simulink model "PTDproj"  (R2016a)
settings: Solver=ode23tb  SolverMode=SingleTasking  StartTime=0.0  StopTime=86400  RelTol=1e-4  AbsTol=1e-3
PreLoadFcn:
  | % Load Data and Parameters used by the model:
  | load power_V2G.mat
  | to=0.1;
undefined symbols (not defined in the file): A, B, C, D1, Dd, Delta, Init, j, V2G
libraries: powerlib x54, simulink x19, simulink_extras x6, sps_avr x1, V2Glib x1, powerlib_meascontrol x1
(part 2 of 3)

== system PTDproj/Scopes /Source data ==
  Complex to Magnitude-Angle : ComplexToMagnitudeAngle
  Complex to Magnitude-Angle1 : ComplexToMagnitudeAngle
  Demux : Demux  Outputs=1
  Demux1 : Demux  Outputs=1
  Gain : Gain  Gain=3/2
  Product : Product
  Product1 : Product
  Product2 : Product
  Sum : Sum  Inputs=|+-
  Trigonometric Function : Trigonometry  Operator=cos
  Trigonometric Function1 : Trigonometry
  V src : Outport
  I src : Outport  Port=2
  S src : Outport  Port=3
  P src : Outport  Port=4
  Q src : Outport  Port=5
  tag scope: P_src=global, Q_src=global, S_src=global
  wires:
  Product2/1 -> [Q_src], Q src/1
  Product1/1 -> P src/1, [P_src]
  Trigonometric Function/1 -> Product1/2
  Trigonometric Function1/1 -> Product2/2
  Sum/1 -> Trigonometric Function/1, Trigonometric Function1/1
  Complex to Magnitude-Angle/2 -> Sum/1
  [Iabc1] -> Complex to Magnitude-Angle1/1
  [Vabc1] -> Complex to Magnitude-Angle/1
  Complex to Magnitude-Angle1/2 -> Sum/2
  Product/1 -> Product1/1, Product2/1, S src/1, [S_src]
  Demux1/1 -> Product/2
  Gain/1 -> Product/1
  Complex to Magnitude-Angle1/1 -> Demux1/1, I src/1
  Complex to Magnitude-Angle/1 -> Demux/1, V src/1
  Demux/1 -> Gain/1

== system PTDproj/Scopes /Wind farm data ==
  Complex to Magnitude-Angle : ComplexToMagnitudeAngle
  Complex to Magnitude-Angle1 : ComplexToMagnitudeAngle
  Demux : Demux  Outputs=1
  Demux1 : Demux  Outputs=1
  Gain : Gain  Gain=3/2
  Product : Product
  Product1 : Product
  Product2 : Product
  Scope : Scope
  Sum : Sum  Inputs=|+-
  Trigonometric Function : Trigonometry  Operator=cos
  Trigonometric Function1 : Trigonometry
  V wind : Outport
  I wind : Outport  Port=2
  S wind : Outport  Port=3
  P wind : Outport  Port=4
  Q wind : Outport  Port=5
  Wind : Outport  Port=6
  tag scope: P_wind=global, Q_wind=global, S_wind=global
  wires:
  Demux/1 -> Gain/1
  Complex to Magnitude-Angle/1 -> V wind/1, Demux/1
  Complex to Magnitude-Angle1/1 -> I wind/1, Demux1/1
  Gain/1 -> Product/1
  Demux1/1 -> Product/2
  Product/1 -> [S_wind], S wind/1, Product2/1, Product1/1
  Complex to Magnitude-Angle1/2 -> Scope/1, Sum/2
  [Vabcwind] -> Complex to Magnitude-Angle/1
  [Iabcwind] -> Complex to Magnitude-Angle1/1
  Complex to Magnitude-Angle/2 -> Sum/1
  Sum/1 -> Trigonometric Function1/1, Trigonometric Function/1
  Trigonometric Function1/1 -> Product2/2
  Trigonometric Function/1 -> Product1/2
  Product1/1 -> [P_wind], P wind/1
  Product2/1 -> [Q_wind], Q wind/1
  [wind] -> Wind/1

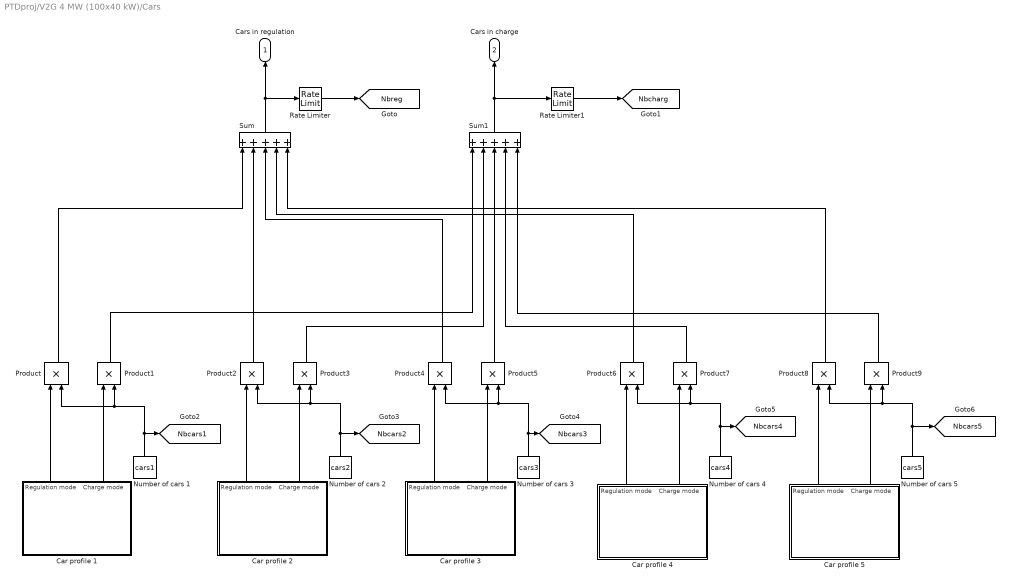
== system PTDproj/V2G 4 MW (100x40 kW)/Cars ==
  Car profile 1 : Subsystem
  Car profile 2 : Subsystem
  Car profile 3 : Subsystem
  Car profile 4 : Subsystem
  Car profile 5 : Subsystem
  Number of cars 1 : Constant  Value=cars1
  Number of cars 2 : Constant  Value=cars2
  Number of cars 3 : Constant  Value=cars3
  Number of cars 4 : Constant  Value=cars4
  Number of cars 5 : Constant  Value=cars5
  Product{,1..9} (10 alike) : Product
  Rate Limiter : RateLimiter  RisingSlewLimit=10000  FallingSlewLimit=-10000  SampleTimeMode=inherited
  Rate Limiter1 : RateLimiter  RisingSlewLimit=10000  FallingSlewLimit=-10000  SampleTimeMode=inherited
  Sum : Sum  Inputs=+++++
  Sum1 : Sum  Inputs=+++++
  Cars in regulation : Outport
  " Cars in charge" : Outport  Port=2
  tag scope: Nbcars1=global, Nbcars2=global, Nbcars3=global, Nbcars4=global, Nbcars5=global, Nbcharg=global, Nbreg=global
  wires:
  Car profile 3/2("Charge mode ") -> Product5/1
  Car profile 2/1("Regulation mode ") -> Product2/1
  Car profile 3/1("Regulation mode ") -> Product4/1
  Car profile 2/2("Charge mode ") -> Product3/1
  Car profile 4/2("Charge mode ") -> Product7/1
  Car profile 4/1("Regulation mode ") -> Product6/1
  Car profile 1/1("Regulation mode ") -> Product/1
  Car profile 1/2("Charge mode ") -> Product1/1
  Number of cars 1/1 -> Product1/2, Product/2, [Nbcars1]
  Number of cars 2/1 -> Product3/2, Product2/2, [Nbcars2]
  Number of cars 3/1 -> Product4/2, Product5/2, [Nbcars3]
  Number of cars 4/1 -> Product6/2, Product7/2, [Nbcars4]
  Number of cars 5/1 -> Product8/2, Product9/2, [Nbcars5]
  Sum/1 -> Cars in regulation/1, Rate Limiter/1
  Sum1/1 -> Rate Limiter1/1, " Cars in charge"/1
  Product/1 -> Sum/1
  Product2/1 -> Sum/2
  Product4/1 -> Sum/3
  Product6/1 -> Sum/4
  Product8/1 -> Sum/5
  Product1/1 -> Sum1/1
  Product3/1 -> Sum1/2
  Product9/1 -> Sum1/5
  Product5/1 -> Sum1/3
  Product7/1 -> Sum1/4
  Rate Limiter/1 -> [Nbreg]
  Rate Limiter1/1 -> [Nbcharg]
  Car profile 5/1("Regulation mode ") -> Product8/1
  Car profile 5/2("Charge mode ") -> Product9/1

== system PTDproj/V2G 4 MW (100x40 kW)/Charge power generation ==
  note: V1= 1/3(Vab -a^2*Vbc)
  note: S = 3* ( V * I') / 2
  note: Ia= I1
  note: Ib= a^2*I1
  S charg : Inport
  Add : Sum  Inputs=+-
  Avoid division by zero : Subsystem
  Break Alg. Loop 2 : Subsystem
  Conj1 : Math  Operator=conj  SaturateOnIntegerOverflow=on
  Demux : Demux  Outputs=2
  Gain : Gain  Gain=-1
  Product : Product  Inputs=/*  SaturateOnIntegerOverflow=on  InputSameDT=on  OutDataTypeStr=Inherit: Same as first input
  Real-Imag to Complex : RealImagToComplex
  a^2 : Gain  Gain=exp(-j*2*pi/3)  SaturateOnIntegerOverflow=on  OutDataTypeStr=Inherit: Same as input  ParamDataTypeStr=Inherit: Same as input
  "a^2 " : Gain  Gain=exp(-j*2*pi/3)  SaturateOnIntegerOverflow=on  OutDataTypeStr=Inherit: Same as input  ParamDataTypeStr=Inherit: Same as input
  a^3 : Gain  Gain=1/3  SaturateOnIntegerOverflow=on  OutDataTypeStr=Inherit: Same as input  ParamDataTypeStr=Inherit: Same as input
  a^4 : Gain  Gain=2/3  SaturateOnIntegerOverflow=on  OutDataTypeStr=Inherit: Same as input  ParamDataTypeStr=Inherit: Same as input
  tag scope: Ia2=global, Ib2=global
  wires:
  Real-Imag to Complex/1 -> Product/2
  Product/1 -> a^4/1  "I1"
  a^2/1 -> [Ib2]
  Avoid division by zero/1(O) -> Product/1  "V1"
  Conj1/1 -> Break Alg. Loop 2/1(In)
  a^3/1 -> Avoid division by zero/1(I)
  Add/1 -> a^3/1
  [Vab2] -> Add/1
  [Vbc2] -> "a^2 "/1
  "a^2 "/1 -> Add/2
  a^4/1 -> Conj1/1
  Break Alg. Loop 2/1(Out) -> [Ia2], a^2/1
  Demux/1 -> Real-Imag to Complex/1
  Demux/2 -> Real-Imag to Complex/2
  S charg/1 -> Gain/1
  Gain/1 -> Demux/1

== system PTDproj/V2G 4 MW (100x40 kW)/Grid regulation ==
  Pmax reg : Inport
  Grid regulation ocntrol : Subsystem
  Grid regulation power  generation : Subsystem
  wires:
  Grid regulation ocntrol/1(PQ) -> Grid regulation power  generation/1("PQ ")
  Pmax reg/1 -> Grid regulation ocntrol/1(Pmax reg)

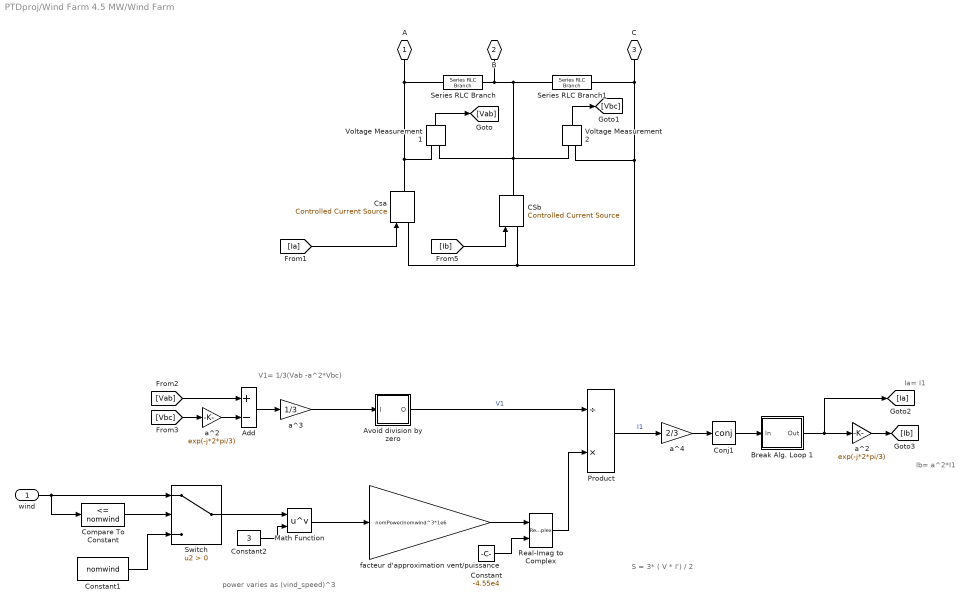
== system PTDproj/Wind Farm 4.5 MW/Wind Farm ==
  note: power varies as (vind_speed)^3
  note: V1= 1/3(Vab -a^2*Vbc)
  note: S = 3* ( V * I') / 2
  note: Ia= I1
  note: Ib= a^2*I1
  "wind " : Inport
  Add : Sum  Inputs=+-
  Avoid division by zero : Subsystem
  Break Alg. Loop 1 : Subsystem
  CSb : powerlib/Electrical Sources/Controlled Current Source  Initialize=on  Source_Type=AC  Amplitude=6286.7  Phase=(-0.5-2*pi/3)*180/pi  Frequency=60  Measurements=Current
  Compare To Constant : simulink/Logic and Bit Operations/Compare To Constant  relop=<=  const=nomwind  OutDataTypeStr=boolean
  Conj1 : Math  Operator=conj  SaturateOnIntegerOverflow=on
  Constant : Constant  Value=-4.55e4
  Constant1 : Constant  Value=nomwind
  Constant2 : Constant  Value=3
  Csa : powerlib/Electrical Sources/Controlled Current Source  Initialize=on  Source_Type=AC  Amplitude=6286.7  Phase=-0.5*180/pi  Frequency=60  Measurements=Current
  Math Function : Math  Operator=pow  SaturateOnIntegerOverflow=on
  Product : Product  Inputs=/*  SaturateOnIntegerOverflow=on  InputSameDT=on  OutDataTypeStr=Inherit: Same as first input
  Real-Imag to Complex : RealImagToComplex
  Series RLC Branch : powerlib/Elements/Series RLC Branch  LConnTagsString=__new0  RConnTagsString=__new0  BranchType=R  Resistance=1e6  Inductance=1e-3  SetiL0=off  InitialCurrent=0  Capacitance=1e-6  Setx0=off  InitialVoltage=0  Measurements=None
  Series RLC Branch1 : powerlib/Elements/Series RLC Branch  LConnTagsString=__new0  RConnTagsString=__new0  BranchType=R  Resistance=1e6  Inductance=1e-3  SetiL0=off  InitialCurrent=0  Capacitance=1e-6  Setx0=off  InitialVoltage=0  Measurements=None
  Switch : Switch  Criteria=u2 > Threshold
  Voltage Measurement1 : powerlib/Measurements/Voltage Measurement  PhasorSimulation=on  OutputType=Complex  PSBequivalent=0
  Voltage Measurement2 : powerlib/Measurements/Voltage Measurement  PhasorSimulation=on  OutputType=Complex  PSBequivalent=0
  a^2 : Gain  Gain=exp(-j*2*pi/3)  SaturateOnIntegerOverflow=on  OutDataTypeStr=Inherit: Same as input  ParamDataTypeStr=Inherit: Same as input
  "a^2 " : Gain  Gain=exp(-j*2*pi/3)  SaturateOnIntegerOverflow=on  OutDataTypeStr=Inherit: Same as input  ParamDataTypeStr=Inherit: Same as input
  a^3 : Gain  Gain=1/3  SaturateOnIntegerOverflow=on  OutDataTypeStr=Inherit: Same as input  ParamDataTypeStr=Inherit: Same as input
  a^4 : Gain  Gain=2/3  SaturateOnIntegerOverflow=on  OutDataTypeStr=Inherit: Same as input  ParamDataTypeStr=Inherit: Same as input
  facteur d'approximation vent/puissance : Gain  Gain=nomPower/nomwind^3*1e6
  A : PMIOPort  Tag=PMCPort  Port=1  Side=Right
  B : PMIOPort  Tag=PMCPort  Port=2  Side=Right
  C : PMIOPort  Tag=PMCPort  Port=3  Side=Right
  wires:
  "a^2 "/1 -> Add/2
  [Vbc] -> "a^2 "/1
  Avoid division by zero/1(O) -> Product/1  "V1"
  a^3/1 -> Avoid division by zero/1(I)
  Add/1 -> a^3/1
  [Vab] -> Add/1
  facteur d'approximation vent/puissance/1 -> Real-Imag to Complex/1
  Constant1/1 -> Switch/3
  Compare To Constant/1 -> Switch/2
  "wind "/1 -> Switch/1, Compare To Constant/1
  Constant/1 -> Real-Imag to Complex/2
  Voltage Measurement1/1 -> [Vab]
  Voltage Measurement2/1 -> [Vbc]
  Real-Imag to Complex/1 -> Product/2
  Product/1 -> a^4/1  "I1"
  a^2/1 -> [Ib]
  Conj1/1 -> Break Alg. Loop 1/1(In)
  a^4/1 -> Conj1/1
  Break Alg. Loop 1/1(Out) -> [Ia], a^2/1
  [Ib] -> CSb/1
  [Ia] -> Csa/1
  Math Function/1 -> facteur d'approximation vent/puissance/1
  Switch/1 -> Math Function/1
  Constant2/1 -> Math Function/2
  connections:
  A/RConn1 -- Csa/RConn1 -- Voltage Measurement1/LConn1 -- Series RLC Branch/LConn1
  Voltage Measurement2/LConn2 -- Series RLC Branch1/RConn1 -- C/RConn1 -- CSb/LConn1 -- Csa/LConn1
  CSb/RConn1 -- Series RLC Branch1/LConn1 -- B/RConn1 -- Series RLC Branch/RConn1 -- Voltage Measurement2/LConn1 -- Voltage Measurement1/LConn2

== system PTDproj/Wind Farm 4.5 MW/Wind control ==
  "wind " : Inport
  Compare To Constant : simulink/Logic and Bit Operations/Compare To Constant  relop=>=  const=maxwind-0.1  OutDataTypeStr=boolean  ZeroCross=off
  Compare To Constant1 : simulink/Logic and Bit Operations/Compare To Constant  relop=<=  const=nomwind  OutDataTypeStr=boolean  ZeroCross=off
  Constant1 : Constant  Value=0
  Constant2 : Constant  Value=9
  Logical Operator1 : Logic  Operator=NOT  AllPortsSameDT=off  OutDataTypeStr=boolean
  Manual Switch : ManualSwitch
  Rate Limiter2 : RateLimiter  RisingSlewLimit=1e4  FallingSlewLimit=-1e4  SampleTimeMode=inherited
  S-R Flip-Flop : simulink_extras/Flip Flops/S-R Flip-Flop  initial_condition=0
  Switch : Switch  Threshold=0.5  ZeroCross=off
  Terminator : Terminator
  Wind : Outport
  wires:
  "wind "/1 -> Switch/1, Compare To Constant/1, Compare To Constant1/1
  Constant1/1 -> Switch/3
  Logical Operator1/1 -> Switch/2
  S-R Flip-Flop/1 -> Logical Operator1/1
  Compare To Constant1/1 -> S-R Flip-Flop/2
  Compare To Constant/1 -> S-R Flip-Flop/1
  S-R Flip-Flop/2 -> Terminator/1
  Switch/1 -> Manual Switch/1
  Manual Switch/1 -> Rate Limiter2/1
  Constant2/1 -> Manual Switch/2
  Rate Limiter2/1 -> Wind/1

== system PTDproj/Load Residential = 10 MW, PF=0.15 ASM = 0.16 MVA /Residential Load/Avoid division by zero ==
  I : Inport
  Complex to Magnitude-Angle : ComplexToMagnitudeAngle
  Magnitude-Angle to Complex : MagnitudeAngleToComplex
  Saturation1 : Saturate  UpperLimit=inf  LowerLimit=1e-6
  O : Outport
  wires:
  I/1 -> Complex to Magnitude-Angle/1
  Saturation1/1 -> Magnitude-Angle to Complex/1
  Complex to Magnitude-Angle/1 -> Saturation1/1
  Magnitude-Angle to Complex/1 -> O/1
  Complex to Magnitude-Angle/2 -> Magnitude-Angle to Complex/2

== system PTDproj/Load Residential = 10 MW, PF=0.15 ASM = 0.16 MVA /Residential Load/Break Alg. Loop 1 ==
  In : Inport
  Complex to Real-Imag : ComplexToRealImag
  Real-Imag to Complex : RealImagToComplex
  imag : Subsystem  mask(Transfer Function with Initial Outputs){N=[1], D=[to  1], Y0=0, U0=0}
      mask prompts: N "Numerator:"; D "Denominator:"; Y0 "Initial output:"; U0 "Initial input:"
      mask help: Vector expressions for numerator, and denominator. Coefficients are in descending powers of s.
      mask init:
      | [A,B,C,Dd]=tf2ss(N,D);if (isempty(Y0));[m,n]=size(A);X0=zeros(1,m); end; if (isempty(U0));[m,p]=size(B);U0=zeros(1,p);end;X0=getxo(A,B,C,Dd,U0,Y0,0);
      mask Help: Specify the initial output for the transfer function.  An optimization routine attempts to determine the appropriate initial states so that the specified initial output is achieved.  For more details, see the m-file getxo.m
      mask Display: dpoly(N,D,'s')
  real : Subsystem  mask(Transfer Function with Initial Outputs){N=[1], D=[to 1], Y0=0, U0=0}
      mask prompts: N "Numerator:"; D "Denominator:"; Y0 "Initial output:"; U0 "Initial input:"
      mask help: Vector expressions for numerator, and denominator. Coefficients are in descending powers of s.
      mask init:
      | [A,B,C,Dd]=tf2ss(N,D);if (isempty(Y0));[m,n]=size(A);X0=zeros(1,m); end; if (isempty(U0));[m,p]=size(B);U0=zeros(1,p);end;X0=getxo(A,B,C,Dd,U0,Y0,0);
      mask Help: Specify the initial output for the transfer function.  An optimization routine attempts to determine the appropriate initial states so that the specified initial output is achieved.  For more details, see the m-file getxo.m
      mask Display: dpoly(N,D,'s')
  Out : Outport
  wires:
  Complex to Real-Imag/1 -> real/1(In1)
  Complex to Real-Imag/2 -> imag/1(In1)
  In/1 -> Complex to Real-Imag/1
  Real-Imag to Complex/1 -> Out/1
  real/1(Out1) -> Real-Imag to Complex/1
  imag/1(Out1) -> Real-Imag to Complex/2

== system PTDproj/Load Residential = 10 MW, PF=0.15 ASM = 0.16 MVA /Residential Load/Load ==
  1 : Constant
  Add : Sum
  Clock : Clock
  Constant : Constant
  Constant1 : Constant  Value=15/24
  Divide : Product  Inputs=*/
  Manual Switch : ManualSwitch
  Mux : Mux  Inputs=2
  P nom : Constant  Value=-nomPower*1e6
  Power consumption : Lookup_n-D  NumberOfTableDimensions=1  BreakpointsForDimension1=[1:timestep/60:24]  BeginIndexSearchUsingPreviousIndexResult=on  Table=datas  InternalRulePriority=Speed  RndMeth=Simplest  InputSameDT=on
  Power factor : Constant  Value=PF^2
  Product : Product
  Product1 : Product
  Scope : Scope
  Second-->Hour : Gain  Gain=1/(60*60)
  Sqrt : Sqrt  SaturateOnIntegerOverflow=on
  Sum : Sum  Inputs=-+
  PQ : Outport
  wires:
  Constant/1 -> Add/2
  1/1 -> Sum/1, Divide/1
  Second-->Hour/1 -> Add/1
  Sum/1 -> Sqrt/1
  Power factor/1 -> Divide/2
  Add/1 -> Power consumption/1
  P nom/1 -> Product/2
  Clock/1 -> Second-->Hour/1
  Sqrt/1 -> Product1/2
  Product/1 -> Product1/1, Mux/1
  Divide/1 -> Sum/2
  Product1/1 -> Mux/2
  Power consumption/1 -> Manual Switch/1
  Manual Switch/1 -> Product/1
  Constant1/1 -> Manual Switch/2
  Mux/1 -> Scope/1, PQ/1

== system PTDproj/PV Farm 8 MW/PV Farm/Avoid division by zero ==
  I : Inport
  Complex to Magnitude-Angle : ComplexToMagnitudeAngle
  Magnitude-Angle to Complex : MagnitudeAngleToComplex
  Saturation1 : Saturate  UpperLimit=inf  LowerLimit=1e-6
  O : Outport
  wires:
  Complex to Magnitude-Angle/2 -> Magnitude-Angle to Complex/2
  Magnitude-Angle to Complex/1 -> O/1
  Complex to Magnitude-Angle/1 -> Saturation1/1
  Saturation1/1 -> Magnitude-Angle to Complex/1
  I/1 -> Complex to Magnitude-Angle/1

== system PTDproj/PV Farm 8 MW/PV Farm/Break Alg. Loop 1 ==
  In : Inport
  Complex to Real-Imag : ComplexToRealImag
  Real-Imag to Complex : RealImagToComplex
  imag : Subsystem  mask(Transfer Function with Initial Outputs){N=[1], D=[to  1], Y0=0, U0=0}
      mask prompts: N "Numerator:"; D "Denominator:"; Y0 "Initial output:"; U0 "Initial input:"
      mask help: Vector expressions for numerator, and denominator. Coefficients are in descending powers of s.
      mask init:
      | [A,B,C,Dd]=tf2ss(N,D);if (isempty(Y0));[m,n]=size(A);X0=zeros(1,m); end; if (isempty(U0));[m,p]=size(B);U0=zeros(1,p);end;X0=getxo(A,B,C,Dd,U0,Y0,0);
      mask Help: Specify the initial output for the transfer function.  An optimization routine attempts to determine the appropriate initial states so that the specified initial output is achieved.  For more details, see the m-file getxo.m
      mask Display: dpoly(N,D,'s')
  real : Subsystem  mask(Transfer Function with Initial Outputs){N=[1], D=[to 1], Y0=0, U0=0}
      mask prompts: N "Numerator:"; D "Denominator:"; Y0 "Initial output:"; U0 "Initial input:"
      mask help: Vector expressions for numerator, and denominator. Coefficients are in descending powers of s.
      mask init:
      | [A,B,C,Dd]=tf2ss(N,D);if (isempty(Y0));[m,n]=size(A);X0=zeros(1,m); end; if (isempty(U0));[m,p]=size(B);U0=zeros(1,p);end;X0=getxo(A,B,C,Dd,U0,Y0,0);
      mask Help: Specify the initial output for the transfer function.  An optimization routine attempts to determine the appropriate initial states so that the specified initial output is achieved.  For more details, see the m-file getxo.m
      mask Display: dpoly(N,D,'s')
  Out : Outport
  wires:
  Complex to Real-Imag/1 -> real/1(In1)
  Complex to Real-Imag/2 -> imag/1(In1)
  In/1 -> Complex to Real-Imag/1
  Real-Imag to Complex/1 -> Out/1
  real/1(Out1) -> Real-Imag to Complex/1
  imag/1(Out1) -> Real-Imag to Complex/2

== system PTDproj/V2G 4 MW (100x40 kW)/Cars/Car profile 1 ==
  Add : Sum
  Charger control : Subsystem
  Clock : Clock
  Constant : Constant
  Plug state : Lookup_n-D  NumberOfTableDimensions=1  BreakpointsForDimension1=[1:24]  BeginIndexSearchUsingPreviousIndexResult=on  Table="[1 1 1 1 1 1 0 0 1 1 1 1 1 1 1 1 0 0 1 1 1 1  1 1]"  InterpMethod=Flat  InternalRulePriority=Speed  RndMeth=Simplest  InputSameDT=on
  Rate Limiter : RateLimiter  RisingSlewLimit=1e4  FallingSlewLimit=-1e4  SampleTimeMode=inherited
  Rate Limiter1 : RateLimiter  RisingSlewLimit=1e4  FallingSlewLimit=-1e4  SampleTimeMode=inherited
  SOC initialization : Lookup_n-D  NumberOfTableDimensions=1  BreakpointsForDimension1=[1:24]  BeginIndexSearchUsingPreviousIndexResult=on  Table=[0.9 0.9 0.9 0.9 0.9 0.9 -1 0.8 0.8 0.9 0.9 0.9 0.9 0.9 0.9 0.9 -1 0.8 0.8 0.9 0.9 0.9 0.9 0.9]  InterpMethod=Flat  InternalRulePriority=Speed  RndMeth=Simplest  InputSameDT=on
  Second-->Hour : Gain  Gain=1/(60*60)
  State of charge : Subsystem
  "Regulation mode " : Outport
  "Charge mode " : Outport  Port=2
  wires:
  Constant/1 -> Add/2
  Second-->Hour/1 -> Add/1
  Clock/1 -> Second-->Hour/1
  Add/1 -> SOC initialization/1, Plug state/1
  State of charge/1(SE%) -> Charger control/1(SE%)
  Charger control/1("Charge mode ") -> "Charge mode "/1, State of charge/1(charge)
  Charger control/2("Regulation mode ") -> "Regulation mode "/1
  SOC initialization/1 -> Rate Limiter/1
  Plug state/1 -> Rate Limiter1/1
  Rate Limiter/1 -> State of charge/2(SOC)
  Rate Limiter1/1 -> Charger control/2("Plug "), State of charge/3(Plug)

== system PTDproj/V2G 4 MW (100x40 kW)/Cars/Car profile 2 ==
  Add1 : Sum
  Charger control : Subsystem
  Clock1 : Clock
  Constant1 : Constant
  Plug state : Lookup_n-D  NumberOfTableDimensions=1  BreakpointsForDimension1=[1:24]  BeginIndexSearchUsingPreviousIndexResult=on  Table="[1 1 1 1 1 1 0 0 0 0 0 0 0 0 0 0 0 0 1 1 1 1  1 1]"  InterpMethod=Flat  InternalRulePriority=Speed  RndMeth=Simplest  InputSameDT=on
  Rate Limiter2 : RateLimiter  RisingSlewLimit=1e4  FallingSlewLimit=-1e4  SampleTimeMode=inherited
  Rate Limiter3 : RateLimiter  RisingSlewLimit=1e4  FallingSlewLimit=-1e4  SampleTimeMode=inherited
  SOC initialization : Lookup_n-D  NumberOfTableDimensions=1  BreakpointsForDimension1=[1:24]  BeginIndexSearchUsingPreviousIndexResult=on  Table=[0.9 0.9 0.9 0.9 0.9 0.9 -1 0.8 0.8 0.9 0.9 0.9 0.9 0.9 0.9 0.9 -1 0.8 0.6 0.9 0.9 0.9 0.9 0.9]  InterpMethod=Flat  InternalRulePriority=Speed  RndMeth=Simplest  InputSameDT=on
  Second-->Hour1 : Gain  Gain=1/(60*60)
  State of charge : Subsystem
  "Regulation mode " : Outport
  "Charge mode " : Outport  Port=2
  wires:
  Constant1/1 -> Add1/2
  Second-->Hour1/1 -> Add1/1
  Clock1/1 -> Second-->Hour1/1
  Add1/1 -> Plug state/1, SOC initialization/1
  State of charge/1(SE%) -> Charger control/1(SE%)
  Charger control/1("Charge mode ") -> State of charge/1(charge), "Charge mode "/1
  Charger control/2("Regulation mode ") -> "Regulation mode "/1
  SOC initialization/1 -> Rate Limiter2/1
  Plug state/1 -> Rate Limiter3/1
  Rate Limiter2/1 -> State of charge/2(SOC)
  Rate Limiter3/1 -> Charger control/2("Plug "), State of charge/3(Plug)

== system PTDproj/V2G 4 MW (100x40 kW)/Cars/Car profile 3 ==
  Add1 : Sum
  Charger control : Subsystem
  Clock1 : Clock
  Constant1 : Constant
  Plug state : Lookup_n-D  NumberOfTableDimensions=1  BreakpointsForDimension1=[1:24]  BeginIndexSearchUsingPreviousIndexResult=on  Table="[1 1 1 1 1 0 0 0 1 1 1 1 1 1 1 1 0 0 0 1 1 1  1 1]"  InterpMethod=Flat  InternalRulePriority=Speed  RndMeth=Simplest  InputSameDT=on
  Rate Limiter2 : RateLimiter  RisingSlewLimit=1e4  FallingSlewLimit=-1e4  SampleTimeMode=inherited
  Rate Limiter3 : RateLimiter  RisingSlewLimit=1e4  FallingSlewLimit=-1e4  SampleTimeMode=inherited
  SOC initialization : Lookup_n-D  NumberOfTableDimensions=1  BreakpointsForDimension1=[1:24]  BeginIndexSearchUsingPreviousIndexResult=on  Table=[0.9 0.9 0.9 0.9 0.9 -1 -1 0.7 0.7 0.9 0.9 0.9 0.9 0.9 0.9 0.9 -1 0.8 0.7 0.9 0.9 0.9 0.9 0.9]  InterpMethod=Flat  InternalRulePriority=Speed  RndMeth=Simplest  InputSameDT=on
  Second-->Hour1 : Gain  Gain=1/(60*60)
  State of charge : Subsystem
  "Regulation mode " : Outport
  "Charge mode " : Outport  Port=2
  wires:
  Constant1/1 -> Add1/2
  Second-->Hour1/1 -> Add1/1
  Clock1/1 -> Second-->Hour1/1
  Add1/1 -> Plug state/1, SOC initialization/1
  Charger control/1("Charge mode ") -> State of charge/1(charge), "Charge mode "/1
  Charger control/2("Regulation mode ") -> "Regulation mode "/1
  SOC initialization/1 -> Rate Limiter2/1
  Plug state/1 -> Rate Limiter3/1
  Rate Limiter2/1 -> State of charge/2(SOC)
  Rate Limiter3/1 -> State of charge/3(Plug), Charger control/2("Plug ")
  State of charge/1(SE%) -> Charger control/1(SE%)

== system PTDproj/V2G 4 MW (100x40 kW)/Cars/Car profile 4 ==
  Add1 : Sum
  Charger control : Subsystem
  Clock1 : Clock
  Constant1 : Constant
  Plug state : Lookup_n-D  NumberOfTableDimensions=1  BreakpointsForDimension1=[1:24]  BeginIndexSearchUsingPreviousIndexResult=on  Table="[1 1 1 1 1 1 1 1 1 1 1 1 1 1 1 1 1 1 1 1 1 1  1 1]"  InterpMethod=Flat  InternalRulePriority=Speed  RndMeth=Simplest  InputSameDT=on
  Rate Limiter2 : RateLimiter  RisingSlewLimit=1e4  FallingSlewLimit=-1e4  SampleTimeMode=inherited
  Rate Limiter3 : RateLimiter  RisingSlewLimit=1e4  FallingSlewLimit=-1e4  SampleTimeMode=inherited
  SOC initialization : Lookup_n-D  NumberOfTableDimensions=1  BreakpointsForDimension1=[1:24]  BeginIndexSearchUsingPreviousIndexResult=on  Table=[0.9 0.9 0.9 0.9 0.9 0.9 0.8 0.8 0.8 0.9 0.9 0.9 0.9 0.9 0.9 0.9 0.8 0.8 0.8 0.9 0.9 0.9 0.9 0.9]  InterpMethod=Flat  InternalRulePriority=Speed  RndMeth=Simplest  InputSameDT=on
  Second-->Hour1 : Gain  Gain=1/(60*60)
  State of charge : Subsystem
  "Regulation mode " : Outport
  "Charge mode " : Outport  Port=2
  wires:
  Constant1/1 -> Add1/2
  Second-->Hour1/1 -> Add1/1
  Clock1/1 -> Second-->Hour1/1
  Add1/1 -> Plug state/1, SOC initialization/1
  State of charge/1(SE%) -> Charger control/1(SE%)
  Charger control/1("Charge mode ") -> State of charge/1(charge), "Charge mode "/1
  Charger control/2("Regulation mode ") -> "Regulation mode "/1
  SOC initialization/1 -> Rate Limiter2/1
  Plug state/1 -> Rate Limiter3/1
  Rate Limiter2/1 -> State of charge/2(SOC)
  Rate Limiter3/1 -> Charger control/2("Plug "), State of charge/3(Plug)

== system PTDproj/V2G 4 MW (100x40 kW)/Cars/Car profile 5 ==
  Add : Sum
  Charger control : Subsystem
  Clock : Clock
  Constant : Constant
  Plug state : Lookup_n-D  NumberOfTableDimensions=1  BreakpointsForDimension1=[1:24]  BeginIndexSearchUsingPreviousIndexResult=on  Table="[0 0 0 0 1 1 1 1 1 1 1 1 1 1 1 1 1 1 1 1 0 0  0 0]"  InterpMethod=Flat  InternalRulePriority=Speed  RndMeth=Simplest  InputSameDT=on
  Rate Limiter : RateLimiter  RisingSlewLimit=1e4  FallingSlewLimit=-1e4  SampleTimeMode=inherited
  Rate Limiter1 : RateLimiter  RisingSlewLimit=1e4  FallingSlewLimit=-1e4  SampleTimeMode=inherited
  SOC initialization : Lookup_n-D  NumberOfTableDimensions=1  BreakpointsForDimension1=[1:24]  BeginIndexSearchUsingPreviousIndexResult=on  Table=[-1 0.9 0.7 0.7 0.7 0.8 0.8 0.8 0.8 0.8 0.9 0.9 0.9 0.9 0.9 0.9 0.8 0.8 0.8 0.9 -1 0.9 0.9 0.9]  InterpMethod=Flat  InternalRulePriority=Speed  RndMeth=Simplest  InputSameDT=on
  Second-->Hour : Gain  Gain=1/(60*60)
  State of charge : Subsystem
  "Regulation mode " : Outport
  "Charge mode " : Outport  Port=2
  wires:
  Rate Limiter1/1 -> State of charge/1(Plug), Charger control/2("Plug ")
  Rate Limiter/1 -> State of charge/2(SOC)
  Plug state/1 -> Rate Limiter1/1
  SOC initialization/1 -> Rate Limiter/1
  Charger control/2("Regulation mode ") -> "Regulation mode "/1
  Charger control/1("Charge mode ") -> "Charge mode "/1, State of charge/3(charge)
  State of charge/1(SE%) -> Charger control/1(SE%)
  Add/1 -> Plug state/1, SOC initialization/1
  Clock/1 -> Second-->Hour/1
  Second-->Hour/1 -> Add/1
  Constant/1 -> Add/2

== system PTDproj/V2G 4 MW (100x40 kW)/Charge power generation/Avoid division by zero ==
  I : Inport
  Complex to Magnitude-Angle : ComplexToMagnitudeAngle
  Magnitude-Angle to Complex : MagnitudeAngleToComplex
  Saturation1 : Saturate  UpperLimit=inf  LowerLimit=1e-6
  O : Outport
  wires:
  I/1 -> Complex to Magnitude-Angle/1
  Saturation1/1 -> Magnitude-Angle to Complex/1
  Complex to Magnitude-Angle/1 -> Saturation1/1
  Magnitude-Angle to Complex/1 -> O/1
  Complex to Magnitude-Angle/2 -> Magnitude-Angle to Complex/2

== system PTDproj/V2G 4 MW (100x40 kW)/Charge power generation/Break Alg. Loop 2 ==
  In : Inport
  Complex to Real-Imag : ComplexToRealImag
  Real-Imag to Complex : RealImagToComplex
  imag : Subsystem  mask(Transfer Function with Initial Outputs){N=[1], D=[to  1], Y0=0, U0=0}
      mask prompts: N "Numerator:"; D "Denominator:"; Y0 "Initial output:"; U0 "Initial input:"
      mask help: Vector expressions for numerator, and denominator. Coefficients are in descending powers of s.
      mask init:
      | [A,B,C,Dd]=tf2ss(N,D);if (isempty(Y0));[m,n]=size(A);X0=zeros(1,m); end; if (isempty(U0));[m,p]=size(B);U0=zeros(1,p);end;X0=getxo(A,B,C,Dd,U0,Y0,0);
      mask Help: Specify the initial output for the transfer function.  An optimization routine attempts to determine the appropriate initial states so that the specified initial output is achieved.  For more details, see the m-file getxo.m
      mask Display: dpoly(N,D,'s')
  real : Subsystem  mask(Transfer Function with Initial Outputs){N=[1], D=[to 1], Y0=0, U0=0}
      mask prompts: N "Numerator:"; D "Denominator:"; Y0 "Initial output:"; U0 "Initial input:"
      mask help: Vector expressions for numerator, and denominator. Coefficients are in descending powers of s.
      mask init:
      | [A,B,C,Dd]=tf2ss(N,D);if (isempty(Y0));[m,n]=size(A);X0=zeros(1,m); end; if (isempty(U0));[m,p]=size(B);U0=zeros(1,p);end;X0=getxo(A,B,C,Dd,U0,Y0,0);
      mask Help: Specify the initial output for the transfer function.  An optimization routine attempts to determine the appropriate initial states so that the specified initial output is achieved.  For more details, see the m-file getxo.m
      mask Display: dpoly(N,D,'s')
  Out : Outport
  wires:
  Complex to Real-Imag/1 -> real/1(In1)
  Complex to Real-Imag/2 -> imag/1(In1)
  In/1 -> Complex to Real-Imag/1
  Real-Imag to Complex/1 -> Out/1
  real/1(Out1) -> Real-Imag to Complex/1
  imag/1(Out1) -> Real-Imag to Complex/2

== system PTDproj/V2G 4 MW (100x40 kW)/Grid regulation/Grid regulation ocntrol ==
  Pmax reg : Inport
  Clock : Clock
  Compare To Constant : simulink/Logic and Bit Operations/Compare To Constant  relop=>=  const=5e-4  OutDataTypeStr=boolean  ZeroCross=off
  Compare To Constant1 : simulink/Logic and Bit Operations/Compare To Constant  relop=<=  const=-5e-4  OutDataTypeStr=boolean  ZeroCross=off
  Compare To Constant2 : simulink/Logic and Bit Operations/Compare To Constant  relop=>  const=1  OutDataTypeStr=boolean  ZeroCross=off
  Derivative : Derivative
  Gain : Gain  Gain=regGain(2)*1e6
  Gain1 : Gain  Gain=regGain(1)*1e6
  Gain2 : Gain  Gain=-1
  Integrator Limited : Integrator  ExternalReset=falling  UpperSaturationLimit=1e6  LowerSaturationLimit=-1e6
  Logical Operator : Logic  Operator=OR  AllPortsSameDT=off  OutDataTypeStr=boolean
  Logical Operator1 : Logic  AllPortsSameDT=off  OutDataTypeStr=boolean
  Mux : Mux  Inputs=2
  Q : Constant  Value=0
  Q1 : Constant  Value=0
  Saturation Dynamic : simulink/Discontinuities/Saturation Dynamic  OutMin=[]  OutMax=[]  OutDataTypeStr=Inherit: Same as second input  OutDataType=fixdt(1, 16)  OutScaling=2^-10  DoSatur=off
  Sum : Sum  Inputs=|+-
  Sum1 : Sum  Inputs=|++
  Switch : Switch  Threshold=0.5  ZeroCross=off
  wref : Constant
  PQ : Outport
  wires:
  Compare To Constant2/1 -> Logical Operator1/2
  Clock/1 -> Compare To Constant2/1
  Logical Operator/1 -> Logical Operator1/1
  Gain2/1 -> Saturation Dynamic/3
  Pmax reg/1 -> Saturation Dynamic/1, Gain2/1
  Integrator Limited/1 -> Saturation Dynamic/2
  Compare To Constant1/1 -> Logical Operator/2
  Compare To Constant/1 -> Logical Operator/1
  Sum/1 -> Compare To Constant/1, Compare To Constant1/1, Switch/1
  Switch/1 -> Derivative/1, Gain/1
  Gain/1 -> Sum1/2
  Gain1/1 -> Sum1/1
  Derivative/1 -> Gain1/1
  Sum1/1 -> Integrator Limited/1
  Q1/1 -> Switch/3
  [wm] -> Sum/2
  wref/1 -> Sum/1
  Q/1 -> Mux/2
  Mux/1 -> PQ/1
  Logical Operator1/1 -> Integrator Limited/2, Switch/2
  Saturation Dynamic/1 -> Mux/1

== system PTDproj/V2G 4 MW (100x40 kW)/Grid regulation/Grid regulation power  generation ==
  note: V1= 1/3(Vab -a^2*Vbc)
  note: S = 3* ( V * I') / 2
  note: Ia= I1
  note: Ib= a^2*I1
  "PQ " : Inport
  Add : Sum  Inputs=+-
  Avoid division by zero : Subsystem
  Break Alg. Loop 1 : Subsystem
  Conj1 : Math  Operator=conj  SaturateOnIntegerOverflow=on
  Demux : Demux  Outputs=2
  Product : Product  Inputs=/*  SaturateOnIntegerOverflow=on  InputSameDT=on  OutDataTypeStr=Inherit: Same as first input
  Real-Imag to Complex : RealImagToComplex
  a^2 : Gain  Gain=exp(-j*2*pi/3)  SaturateOnIntegerOverflow=on  OutDataTypeStr=Inherit: Same as input  ParamDataTypeStr=Inherit: Same as input
  "a^2 " : Gain  Gain=exp(-j*2*pi/3)  SaturateOnIntegerOverflow=on  OutDataTypeStr=Inherit: Same as input  ParamDataTypeStr=Inherit: Same as input
  a^3 : Gain  Gain=1/3  SaturateOnIntegerOverflow=on  OutDataTypeStr=Inherit: Same as input  ParamDataTypeStr=Inherit: Same as input
  a^4 : Gain  Gain=2/3  SaturateOnIntegerOverflow=on  OutDataTypeStr=Inherit: Same as input  ParamDataTypeStr=Inherit: Same as input
  tag scope: Ia1=global, Ib1=global
  wires:
  Real-Imag to Complex/1 -> Product/2
  Product/1 -> a^4/1  "I1"
  Avoid division by zero/1(O) -> Product/1  "V1"
  Conj1/1 -> Break Alg. Loop 1/1(In)
  a^3/1 -> Avoid division by zero/1(I)
  Add/1 -> a^3/1
  [Vab1] -> Add/1
  [Vbc1] -> "a^2 "/1
  "a^2 "/1 -> Add/2
  a^4/1 -> Conj1/1
  Break Alg. Loop 1/1(Out) -> [Ia1], a^2/1
  Demux/1 -> Real-Imag to Complex/1
  Demux/2 -> Real-Imag to Complex/2
  "PQ "/1 -> Demux/1
  a^2/1 -> [Ib1]

== system PTDproj/Wind Farm 4.5 MW/Wind Farm/Avoid division by zero ==
  I : Inport
  Complex to Magnitude-Angle : ComplexToMagnitudeAngle
  Magnitude-Angle to Complex : MagnitudeAngleToComplex
  Saturation1 : Saturate  UpperLimit=inf  LowerLimit=1e-6
  O : Outport
  wires:
  I/1 -> Complex to Magnitude-Angle/1
  Saturation1/1 -> Magnitude-Angle to Complex/1
  Complex to Magnitude-Angle/1 -> Saturation1/1
  Magnitude-Angle to Complex/1 -> O/1
  Complex to Magnitude-Angle/2 -> Magnitude-Angle to Complex/2

== system PTDproj/Wind Farm 4.5 MW/Wind Farm/Break Alg. Loop 1 ==
  In : Inport
  Complex to Real-Imag : ComplexToRealImag
  Real-Imag to Complex : RealImagToComplex
  imag : Subsystem  mask(Transfer Function with Initial Outputs){N=[1], D=[to  1], Y0=0, U0=0}
      mask prompts: N "Numerator:"; D "Denominator:"; Y0 "Initial output:"; U0 "Initial input:"
      mask help: Vector expressions for numerator, and denominator. Coefficients are in descending powers of s.
      mask init:
      | [A,B,C,Dd]=tf2ss(N,D);if (isempty(Y0));[m,n]=size(A);X0=zeros(1,m); end; if (isempty(U0));[m,p]=size(B);U0=zeros(1,p);end;X0=getxo(A,B,C,Dd,U0,Y0,0);
      mask Help: Specify the initial output for the transfer function.  An optimization routine attempts to determine the appropriate initial states so that the specified initial output is achieved.  For more details, see the m-file getxo.m
      mask Display: dpoly(N,D,'s')
  real : Subsystem  mask(Transfer Function with Initial Outputs){N=[1], D=[to 1], Y0=0, U0=0}
      mask prompts: N "Numerator:"; D "Denominator:"; Y0 "Initial output:"; U0 "Initial input:"
      mask help: Vector expressions for numerator, and denominator. Coefficients are in descending powers of s.
      mask init:
      | [A,B,C,Dd]=tf2ss(N,D);if (isempty(Y0));[m,n]=size(A);X0=zeros(1,m); end; if (isempty(U0));[m,p]=size(B);U0=zeros(1,p);end;X0=getxo(A,B,C,Dd,U0,Y0,0);
      mask Help: Specify the initial output for the transfer function.  An optimization routine attempts to determine the appropriate initial states so that the specified initial output is achieved.  For more details, see the m-file getxo.m
      mask Display: dpoly(N,D,'s')
  Out : Outport
  wires:
  In/1 -> Complex to Real-Imag/1
  Real-Imag to Complex/1 -> Out/1
  real/1(Out1) -> Real-Imag to Complex/1
  imag/1(Out1) -> Real-Imag to Complex/2
  Complex to Real-Imag/2 -> imag/1(In1)
  Complex to Real-Imag/1 -> real/1(In1)

== system PTDproj/Load Residential = 10 MW, PF=0.15 ASM = 0.16 MVA /Residential Load/Break Alg. Loop 1/imag ==
  In1 : Inport
  State Space : StateSpace  A=A  B=B  C=C  D=Dd  X0=X0
  Out1 : Outport  InitialOutput=0
  wires:
  State Space/1 -> Out1/1
  In1/1 -> State Space/1

== system PTDproj/Load Residential = 10 MW, PF=0.15 ASM = 0.16 MVA /Residential Load/Break Alg. Loop 1/real ==
  In1 : Inport
  State Space : StateSpace  A=A  B=B  C=C  D=Dd  X0=X0
  Out1 : Outport  InitialOutput=0
  wires:
  State Space/1 -> Out1/1
  In1/1 -> State Space/1

== system PTDproj/PV Farm 8 MW/PV Farm/Break Alg. Loop 1/imag ==
  In1 : Inport
  State Space : StateSpace  A=A  B=B  C=C  D=Dd  X0=X0
  Out1 : Outport  InitialOutput=0
  wires:
  State Space/1 -> Out1/1
  In1/1 -> State Space/1

== system PTDproj/PV Farm 8 MW/PV Farm/Break Alg. Loop 1/real ==
  In1 : Inport
  State Space : StateSpace  A=A  B=B  C=C  D=Dd  X0=X0
  Out1 : Outport  InitialOutput=0
  wires:
  State Space/1 -> Out1/1
  In1/1 -> State Space/1

== system PTDproj/V2G 4 MW (100x40 kW)/Cars/Car profile 1/Charger control ==
  SE% : Inport
  "Plug " : Inport  Port=2
  Compare To Constant : simulink/Logic and Bit Operations/Compare To Constant  relop=<=  const=85  OutDataTypeStr=boolean  ZeroCross=off
  Compare To Constant1 : simulink/Logic and Bit Operations/Compare To Constant  relop=>=  const=95  OutDataTypeStr=boolean  ZeroCross=off
  Logical Operator : Logic  AllPortsSameDT=off  OutDataTypeStr=boolean
  Logical Operator1 : Logic  Operator=NOT  AllPortsSameDT=off  OutDataTypeStr=boolean
  Logical Operator2 : Logic  AllPortsSameDT=off  OutDataTypeStr=boolean
  S-R Flip-Flop : simulink_extras/Flip Flops/S-R Flip-Flop  initial_condition=0
  Terminator : Terminator
  "Charge mode " : Outport
  "Regulation mode " : Outport  Port=2
  wires:
  SE%/1 -> Compare To Constant/1, Compare To Constant1/1
  Compare To Constant/1 -> S-R Flip-Flop/1
  Compare To Constant1/1 -> S-R Flip-Flop/2
  "Plug "/1 -> Logical Operator2/2, Logical Operator/2
  S-R Flip-Flop/1 -> Logical Operator/1, Logical Operator1/1
  Logical Operator/1 -> "Charge mode "/1
  Logical Operator2/1 -> "Regulation mode "/1
  Logical Operator1/1 -> Logical Operator2/1
  S-R Flip-Flop/2 -> Terminator/1

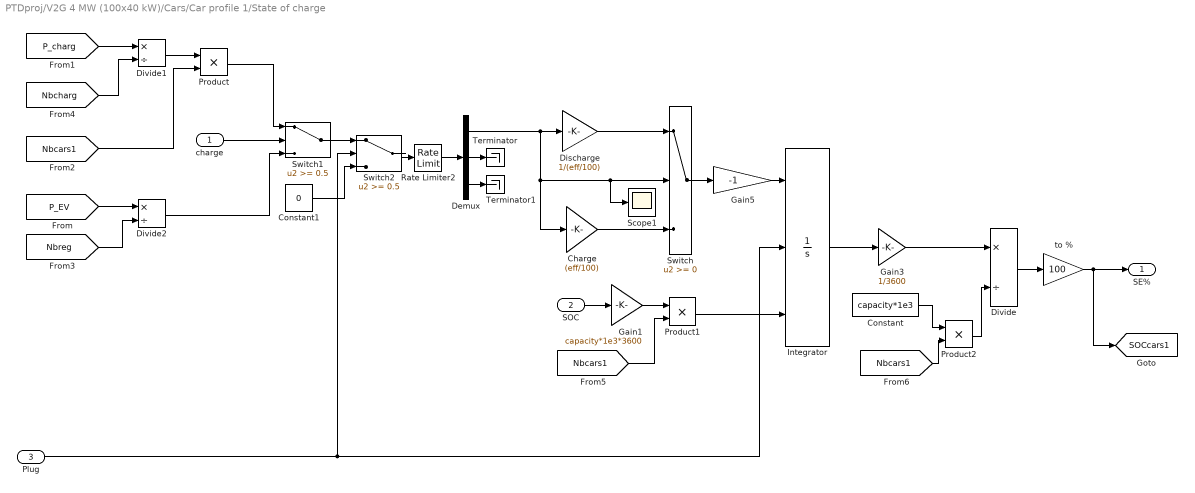
== system PTDproj/V2G 4 MW (100x40 kW)/Cars/Car profile 1/State of charge ==
  charge : Inport
  SOC : Inport  Port=2
  Plug : Inport  Port=3
  Charge : Gain  Gain=(eff/100)
  Constant : Constant  Value=capacity*1e3
  Constant1 : Constant  Value=0
  Demux : Demux  Outputs=3
  Discharge : Gain  Gain=1/(eff/100)
  Divide : Product  Inputs=*/
  Divide1 : Product  Inputs=*/
  Divide2 : Product  Inputs=*/
  Gain1 : Gain  Gain=capacity*1e3*3600
  Gain3 : Gain  Gain=1/3600
  Gain5 : Gain  Gain=-1
  Integrator : Integrator  ExternalReset=either  InitialConditionSource=external  InitialCondition=Init*850e3*3600
  Product : Product
  Product1 : Product
  Product2 : Product
  Rate Limiter2 : RateLimiter  RisingSlewLimit=1e4  FallingSlewLimit=-1e4  SampleTimeMode=inherited
  Scope1 : Scope
  Switch : Switch  ZeroCross=off
  Switch1 : Switch  Threshold=0.5  ZeroCross=off
  Switch2 : Switch  Threshold=0.5  ZeroCross=off
  Terminator : Terminator
  Terminator1 : Terminator
  to % : Gain  Gain=100
  SE% : Outport
  tag scope: SOCcars1=global
  wires:
  Discharge/1 -> Switch/1
  Charge/1 -> Switch/3
  Switch/1 -> Gain5/1
  Gain5/1 -> Integrator/1
  Integrator/1 -> Gain3/1
  Divide/1 -> to %/1
  Gain3/1 -> Divide/1
  to %/1 -> [SOCcars1], SE%/1
  Demux/2 -> Terminator/1
  Demux/3 -> Terminator1/1
  Plug/1 -> Integrator/2, Switch2/2
  SOC/1 -> Gain1/1
  charge/1 -> Switch1/2
  Demux/1 -> Charge/1, Scope1/1, Switch/2, Discharge/1
  [P_charg] -> Divide1/1
  [Nbreg] -> Divide2/2
  [P_EV] -> Divide2/1
  [Nbcharg] -> Divide1/2
  Divide1/1 -> Product/1
  [Nbcars1] -> Product/2
  Product/1 -> Switch1/1
  Divide2/1 -> Switch1/3
  Switch1/1 -> Switch2/1
  Constant1/1 -> Switch2/3
  Switch2/1 -> Rate Limiter2/1
  [Nbcars1] -> Product1/2
  Gain1/1 -> Product1/1
  Product1/1 -> Integrator/3
  Product2/1 -> Divide/2
  [Nbcars1] -> Product2/2
  Constant/1 -> Product2/1
  Rate Limiter2/1 -> Demux/1

== system PTDproj/V2G 4 MW (100x40 kW)/Cars/Car profile 2/Charger control ==
  SE% : Inport
  "Plug " : Inport  Port=2
  Compare To Constant : simulink/Logic and Bit Operations/Compare To Constant  relop=<=  const=85  OutDataTypeStr=boolean  ZeroCross=off
  Compare To Constant1 : simulink/Logic and Bit Operations/Compare To Constant  relop=>=  const=95  OutDataTypeStr=boolean  ZeroCross=off
  Logical Operator : Logic  AllPortsSameDT=off  OutDataTypeStr=boolean
  Logical Operator1 : Logic  Operator=NOT  AllPortsSameDT=off  OutDataTypeStr=boolean
  Logical Operator2 : Logic  AllPortsSameDT=off  OutDataTypeStr=boolean
  S-R Flip-Flop : simulink_extras/Flip Flops/S-R Flip-Flop  initial_condition=0
  Terminator : Terminator
  "Charge mode " : Outport
  "Regulation mode " : Outport  Port=2
  wires:
  SE%/1 -> Compare To Constant/1, Compare To Constant1/1
  Compare To Constant/1 -> S-R Flip-Flop/1
  Compare To Constant1/1 -> S-R Flip-Flop/2
  "Plug "/1 -> Logical Operator2/2, Logical Operator/2
  S-R Flip-Flop/1 -> Logical Operator/1, Logical Operator1/1
  Logical Operator/1 -> "Charge mode "/1
  Logical Operator2/1 -> "Regulation mode "/1
  Logical Operator1/1 -> Logical Operator2/1
  S-R Flip-Flop/2 -> Terminator/1

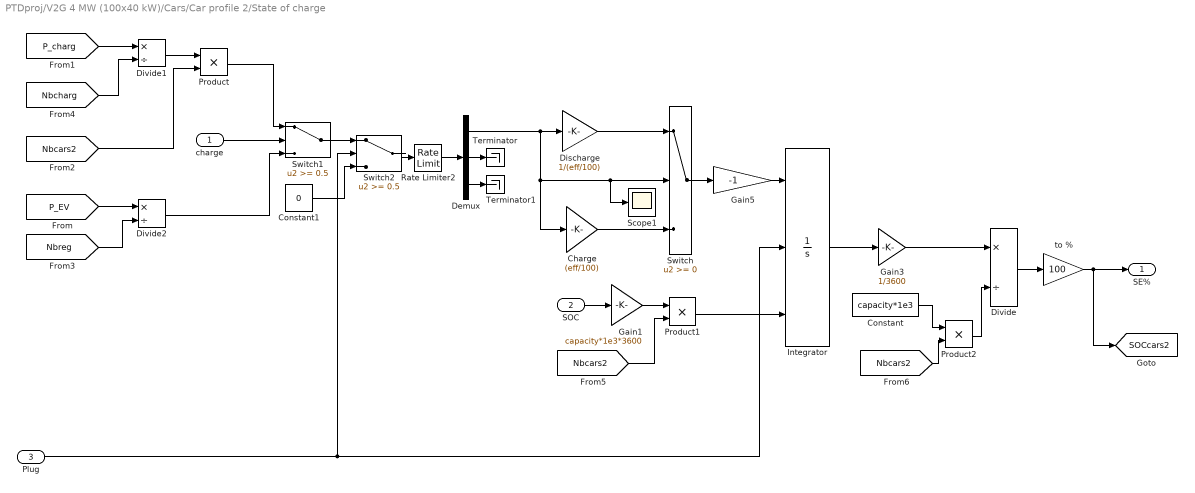
== system PTDproj/V2G 4 MW (100x40 kW)/Cars/Car profile 2/State of charge ==
  charge : Inport
  SOC : Inport  Port=2
  Plug : Inport  Port=3
  Charge : Gain  Gain=(eff/100)
  Constant : Constant  Value=capacity*1e3
  Constant1 : Constant  Value=0
  Demux : Demux  Outputs=3
  Discharge : Gain  Gain=1/(eff/100)
  Divide : Product  Inputs=*/
  Divide1 : Product  Inputs=*/
  Divide2 : Product  Inputs=*/
  Gain1 : Gain  Gain=capacity*1e3*3600
  Gain3 : Gain  Gain=1/3600
  Gain5 : Gain  Gain=-1
  Integrator : Integrator  ExternalReset=either  InitialConditionSource=external  InitialCondition=Init*850e3*3600
  Product : Product
  Product1 : Product
  Product2 : Product
  Rate Limiter2 : RateLimiter  RisingSlewLimit=1e4  FallingSlewLimit=-1e4  SampleTimeMode=inherited
  Scope1 : Scope
  Switch : Switch  ZeroCross=off
  Switch1 : Switch  Threshold=0.5  ZeroCross=off
  Switch2 : Switch  Threshold=0.5  ZeroCross=off
  Terminator : Terminator
  Terminator1 : Terminator
  to % : Gain  Gain=100
  SE% : Outport
  tag scope: SOCcars2=global
  wires:
  Discharge/1 -> Switch/1
  Charge/1 -> Switch/3
  Switch/1 -> Gain5/1
  Gain5/1 -> Integrator/1
  Integrator/1 -> Gain3/1
  Divide/1 -> to %/1
  Gain3/1 -> Divide/1
  to %/1 -> [SOCcars2], SE%/1
  Demux/2 -> Terminator/1
  Demux/3 -> Terminator1/1
  Plug/1 -> Integrator/2, Switch2/2
  SOC/1 -> Gain1/1
  charge/1 -> Switch1/2
  Demux/1 -> Charge/1, Scope1/1, Switch/2, Discharge/1
  [P_charg] -> Divide1/1
  [Nbreg] -> Divide2/2
  [P_EV] -> Divide2/1
  [Nbcharg] -> Divide1/2
  Divide1/1 -> Product/1
  [Nbcars2] -> Product/2
  Product/1 -> Switch1/1
  Divide2/1 -> Switch1/3
  Switch1/1 -> Switch2/1
  Constant1/1 -> Switch2/3
  Switch2/1 -> Rate Limiter2/1
  [Nbcars2] -> Product1/2
  Gain1/1 -> Product1/1
  Product1/1 -> Integrator/3
  Product2/1 -> Divide/2
  [Nbcars2] -> Product2/2
  Constant/1 -> Product2/1
  Rate Limiter2/1 -> Demux/1

== system PTDproj/V2G 4 MW (100x40 kW)/Cars/Car profile 3/Charger control ==
  SE% : Inport
  "Plug " : Inport  Port=2
  Compare To Constant : simulink/Logic and Bit Operations/Compare To Constant  relop=<=  const=85  OutDataTypeStr=boolean  ZeroCross=off
  Compare To Constant1 : simulink/Logic and Bit Operations/Compare To Constant  relop=>=  const=95  OutDataTypeStr=boolean  ZeroCross=off
  Logical Operator : Logic  AllPortsSameDT=off  OutDataTypeStr=boolean
  Logical Operator1 : Logic  Operator=NOT  AllPortsSameDT=off  OutDataTypeStr=boolean
  Logical Operator2 : Logic  AllPortsSameDT=off  OutDataTypeStr=boolean
  S-R Flip-Flop : simulink_extras/Flip Flops/S-R Flip-Flop  initial_condition=0
  Terminator : Terminator
  "Charge mode " : Outport
  "Regulation mode " : Outport  Port=2
  wires:
  SE%/1 -> Compare To Constant/1, Compare To Constant1/1
  Compare To Constant/1 -> S-R Flip-Flop/1
  Compare To Constant1/1 -> S-R Flip-Flop/2
  "Plug "/1 -> Logical Operator2/2, Logical Operator/2
  S-R Flip-Flop/1 -> Logical Operator/1, Logical Operator1/1
  Logical Operator/1 -> "Charge mode "/1
  Logical Operator2/1 -> "Regulation mode "/1
  Logical Operator1/1 -> Logical Operator2/1
  S-R Flip-Flop/2 -> Terminator/1

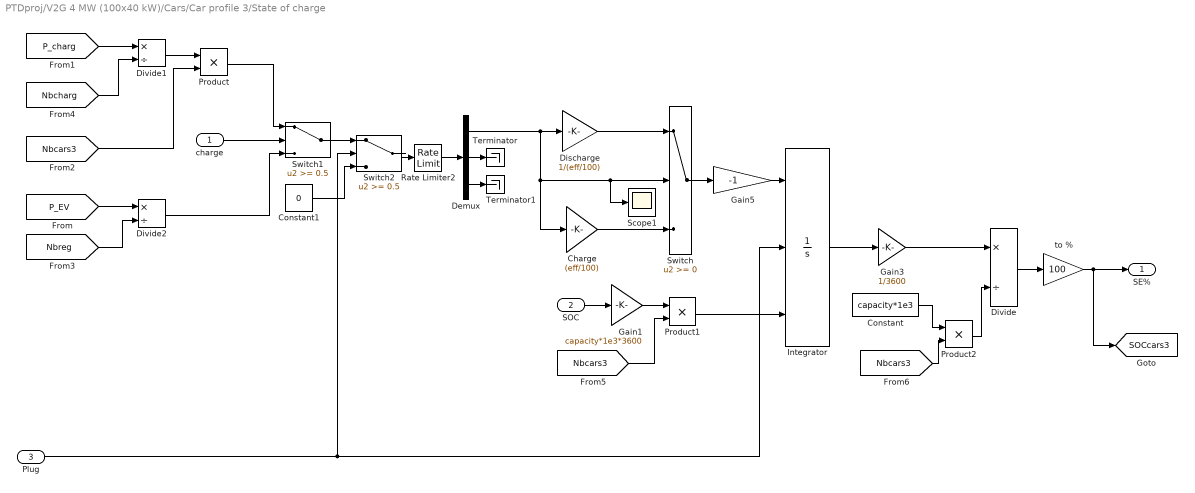
== system PTDproj/V2G 4 MW (100x40 kW)/Cars/Car profile 3/State of charge ==
  charge : Inport
  SOC : Inport  Port=2
  Plug : Inport  Port=3
  Charge : Gain  Gain=(eff/100)
  Constant : Constant  Value=capacity*1e3
  Constant1 : Constant  Value=0
  Demux : Demux  Outputs=3
  Discharge : Gain  Gain=1/(eff/100)
  Divide : Product  Inputs=*/
  Divide1 : Product  Inputs=*/
  Divide2 : Product  Inputs=*/
  Gain1 : Gain  Gain=capacity*1e3*3600
  Gain3 : Gain  Gain=1/3600
  Gain5 : Gain  Gain=-1
  Integrator : Integrator  ExternalReset=either  InitialConditionSource=external  InitialCondition=Init*850e3*3600
  Product : Product
  Product1 : Product
  Product2 : Product
  Rate Limiter2 : RateLimiter  RisingSlewLimit=1e4  FallingSlewLimit=-1e4  SampleTimeMode=inherited
  Scope1 : Scope
  Switch : Switch  ZeroCross=off
  Switch1 : Switch  Threshold=0.5  ZeroCross=off
  Switch2 : Switch  Threshold=0.5  ZeroCross=off
  Terminator : Terminator
  Terminator1 : Terminator
  to % : Gain  Gain=100
  SE% : Outport
  tag scope: SOCcars3=global
  wires:
  Discharge/1 -> Switch/1
  Charge/1 -> Switch/3
  Switch/1 -> Gain5/1
  Gain5/1 -> Integrator/1
  Integrator/1 -> Gain3/1
  Divide/1 -> to %/1
  Gain3/1 -> Divide/1
  to %/1 -> [SOCcars3], SE%/1
  Demux/2 -> Terminator/1
  Demux/3 -> Terminator1/1
  Plug/1 -> Integrator/2, Switch2/2
  SOC/1 -> Gain1/1
  charge/1 -> Switch1/2
  Demux/1 -> Charge/1, Scope1/1, Switch/2, Discharge/1
  [P_charg] -> Divide1/1
  [Nbreg] -> Divide2/2
  [P_EV] -> Divide2/1
  [Nbcharg] -> Divide1/2
  Divide1/1 -> Product/1
  [Nbcars3] -> Product/2
  Product/1 -> Switch1/1
  Divide2/1 -> Switch1/3
  Switch1/1 -> Switch2/1
  Constant1/1 -> Switch2/3
  Switch2/1 -> Rate Limiter2/1
  [Nbcars3] -> Product1/2
  Gain1/1 -> Product1/1
  Product1/1 -> Integrator/3
  Product2/1 -> Divide/2
  [Nbcars3] -> Product2/2
  Constant/1 -> Product2/1
  Rate Limiter2/1 -> Demux/1

== system PTDproj/V2G 4 MW (100x40 kW)/Cars/Car profile 4/Charger control ==
  SE% : Inport
  "Plug " : Inport  Port=2
  Compare To Constant : simulink/Logic and Bit Operations/Compare To Constant  relop=<=  const=85  OutDataTypeStr=boolean  ZeroCross=off
  Compare To Constant1 : simulink/Logic and Bit Operations/Compare To Constant  relop=>=  const=95  OutDataTypeStr=boolean  ZeroCross=off
  Logical Operator : Logic  AllPortsSameDT=off  OutDataTypeStr=boolean
  Logical Operator1 : Logic  Operator=NOT  AllPortsSameDT=off  OutDataTypeStr=boolean
  Logical Operator2 : Logic  AllPortsSameDT=off  OutDataTypeStr=boolean
  S-R Flip-Flop : simulink_extras/Flip Flops/S-R Flip-Flop  initial_condition=0
  Terminator : Terminator
  "Charge mode " : Outport
  "Regulation mode " : Outport  Port=2
  wires:
  SE%/1 -> Compare To Constant/1, Compare To Constant1/1
  Compare To Constant/1 -> S-R Flip-Flop/1
  Compare To Constant1/1 -> S-R Flip-Flop/2
  "Plug "/1 -> Logical Operator2/2, Logical Operator/2
  S-R Flip-Flop/1 -> Logical Operator/1, Logical Operator1/1
  Logical Operator/1 -> "Charge mode "/1
  Logical Operator2/1 -> "Regulation mode "/1
  Logical Operator1/1 -> Logical Operator2/1
  S-R Flip-Flop/2 -> Terminator/1

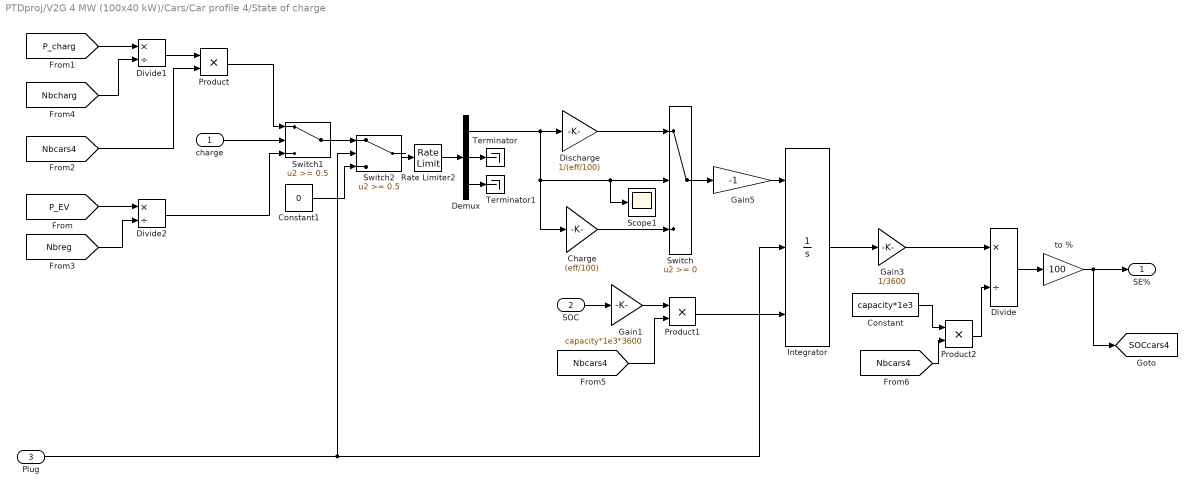
== system PTDproj/V2G 4 MW (100x40 kW)/Cars/Car profile 4/State of charge ==
  charge : Inport
  SOC : Inport  Port=2
  Plug : Inport  Port=3
  Charge : Gain  Gain=(eff/100)
  Constant : Constant  Value=capacity*1e3
  Constant1 : Constant  Value=0
  Demux : Demux  Outputs=3
  Discharge : Gain  Gain=1/(eff/100)
  Divide : Product  Inputs=*/
  Divide1 : Product  Inputs=*/
  Divide2 : Product  Inputs=*/
  Gain1 : Gain  Gain=capacity*1e3*3600
  Gain3 : Gain  Gain=1/3600
  Gain5 : Gain  Gain=-1
  Integrator : Integrator  ExternalReset=either  InitialConditionSource=external  InitialCondition=Init*850e3*3600
  Product : Product
  Product1 : Product
  Product2 : Product
  Rate Limiter2 : RateLimiter  RisingSlewLimit=1e4  FallingSlewLimit=-1e4  SampleTimeMode=inherited
  Scope1 : Scope
  Switch : Switch  ZeroCross=off
  Switch1 : Switch  Threshold=0.5  ZeroCross=off
  Switch2 : Switch  Threshold=0.5  ZeroCross=off
  Terminator : Terminator
  Terminator1 : Terminator
  to % : Gain  Gain=100
  SE% : Outport
  tag scope: SOCcars4=global
  wires:
  Discharge/1 -> Switch/1
  Charge/1 -> Switch/3
  Switch/1 -> Gain5/1
  Gain5/1 -> Integrator/1
  Integrator/1 -> Gain3/1
  Divide/1 -> to %/1
  Gain3/1 -> Divide/1
  to %/1 -> [SOCcars4], SE%/1
  Demux/2 -> Terminator/1
  Demux/3 -> Terminator1/1
  Plug/1 -> Integrator/2, Switch2/2
  SOC/1 -> Gain1/1
  charge/1 -> Switch1/2
  Demux/1 -> Charge/1, Scope1/1, Switch/2, Discharge/1
  [P_charg] -> Divide1/1
  [Nbreg] -> Divide2/2
  [P_EV] -> Divide2/1
  [Nbcharg] -> Divide1/2
  Divide1/1 -> Product/1
  [Nbcars4] -> Product/2
  Product/1 -> Switch1/1
  Divide2/1 -> Switch1/3
  Switch1/1 -> Switch2/1
  Constant1/1 -> Switch2/3
  Switch2/1 -> Rate Limiter2/1
  [Nbcars4] -> Product1/2
  Gain1/1 -> Product1/1
  Product1/1 -> Integrator/3
  Product2/1 -> Divide/2
  [Nbcars4] -> Product2/2
  Constant/1 -> Product2/1
  Rate Limiter2/1 -> Demux/1

== system PTDproj/V2G 4 MW (100x40 kW)/Cars/Car profile 5/Charger control ==
  SE% : Inport
  "Plug " : Inport  Port=2
  Compare To Constant : simulink/Logic and Bit Operations/Compare To Constant  relop=<=  const=85  OutDataTypeStr=boolean
  Compare To Constant1 : simulink/Logic and Bit Operations/Compare To Constant  relop=>=  const=95  OutDataTypeStr=boolean
  Logical Operator : Logic  AllPortsSameDT=off  OutDataTypeStr=boolean
  Logical Operator1 : Logic  Operator=NOT  AllPortsSameDT=off  OutDataTypeStr=boolean
  Logical Operator2 : Logic  AllPortsSameDT=off  OutDataTypeStr=boolean
  S-R Flip-Flop : simulink_extras/Flip Flops/S-R Flip-Flop  initial_condition=0
  Terminator : Terminator
  "Charge mode " : Outport
  "Regulation mode " : Outport  Port=2
  wires:
  S-R Flip-Flop/2 -> Terminator/1
  Logical Operator1/1 -> Logical Operator2/1
  Logical Operator2/1 -> "Regulation mode "/1
  Logical Operator/1 -> "Charge mode "/1
  S-R Flip-Flop/1 -> Logical Operator/1, Logical Operator1/1
  "Plug "/1 -> Logical Operator/2, Logical Operator2/2
  Compare To Constant1/1 -> S-R Flip-Flop/2
  Compare To Constant/1 -> S-R Flip-Flop/1
  SE%/1 -> Compare To Constant/1, Compare To Constant1/1
